simulink model "PID_2DOF"  (Simulink 7.0)
settings: Solver=ode3  StartTime=0.0  StopTime=10.0  RelTol=1e-3
undefined symbols (not defined in the file): Kd1, Kd2, Ki1, Ki2, Kp1, Kp2, L1, L2, M1, M2, theta1, theta2
settings Model: Creator=user  LastModifiedBy=user

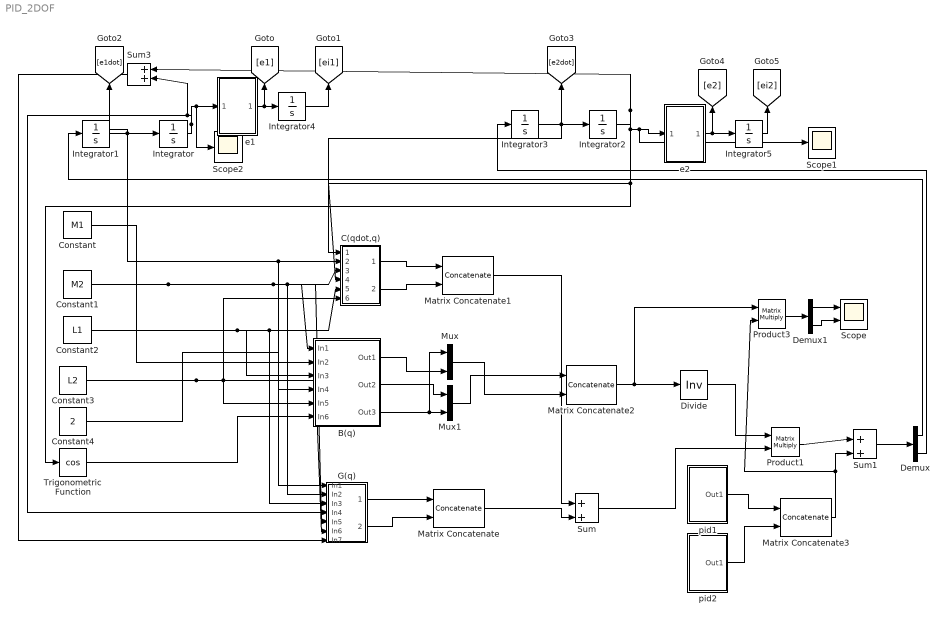
== system PID_2DOF ==
  B(q) : Subsystem
  C(qdot,q) : Subsystem
  Constant : Constant  Value=M1  OutDataType=sfix(16)  OutScaling=2^0
  Constant1 : Constant  Value=M2  OutDataType=sfix(16)  OutScaling=2^0
  Constant2 : Constant  Value=L1  OutDataType=sfix(16)  OutScaling=2^0
  Constant3 : Constant  Value=L2  OutDataType=sfix(16)  OutScaling=2^0
  Constant4 : Constant  Value=2  OutDataType=sfix(16)  OutScaling=2^0
  Demux : Demux  Outputs=2
  Demux1 : Demux  Outputs=2
  Divide : Product  Inputs=/  Multiplication=Matrix(*)  OutDataType=sfix(16)  OutScaling=2^-10
  G(q) : Subsystem
  Integrator{,1..5} (6 alike) : Integrator
  Matrix Concatenate : Concatenate  Mode=Vector  ConcatenateDimension=2
  Matrix Concatenate1 : Concatenate  Mode=Vector  ConcatenateDimension=2
  Matrix Concatenate2 : Concatenate  Mode=Multidimensional array  ConcatenateDimension=2
  Matrix Concatenate3 : Concatenate  Mode=Vector  ConcatenateDimension=2
  Mux : Mux  Inputs=2
  Mux1 : Mux  Inputs=2
  Product1 : Product  Multiplication=Matrix(*)  OutDataType=sfix(16)  OutScaling=2^0  RndMeth=Zero
  Product3 : Product  Multiplication=Matrix(*)  OutDataType=sfix(16)  OutScaling=2^0  RndMeth=Zero
  Scope : Scope  NumInputPorts=2
      settings: YMin=-5~-5  YMax=5~5
  Scope1 : Scope
  Scope2 : Scope
      settings: SaveName=ScopeData2
  Sum : Sum  Inputs=|++  OutDataType=sfix(16)  OutScaling=2^0
  Sum1 : Sum  Inputs=|++  OutDataType=sfix(16)  OutScaling=2^0
  Sum3 : Sum  Orientation=left  Inputs=|++  OutDataType=sfix(16)  OutScaling=2^0
  Trigonometric Function : Trigonometry  Operator=cos
  e1 : Subsystem
  e2 : Subsystem
  pid1 : Subsystem
  pid2 : Subsystem
  wires:
  Constant/1 -> B(q)/2(In2)
  Constant4/1 -> B(q)/4(In4)
  Constant1/1 -> B(q)/1(In1), C(qdot,q)/3(In3), G(q)/2(In2), G(q)/5(In5)
  Constant2/1 -> B(q)/3(In3), C(qdot,q)/5(In5), G(q)/3(In3)
  Constant3/1 -> B(q)/5(In5), C(qdot,q)/6(In6), G(q)/6(In6)
  Trigonometric Function/1 -> B(q)/6(In6)
  Integrator1/1 -> Integrator/1, C(qdot,q)/2(In2), G(q)/1(In1), [e1dot]
  Integrator3/1 -> Integrator2/1, C(qdot,q)/1(In1), [e2dot]
  Integrator2/1 -> Trigonometric Function/1, C(qdot,q)/4(In4), Sum3/1, e2/1(In1), Scope1/1
  Integrator/1 -> Sum3/2, G(q)/4(In4), e1/1(In1), Scope2/1
  Sum3/1 -> G(q)/7(In7)
  G(q)/1(Out1) -> Matrix Concatenate/1
  G(q)/2(Out2) -> Matrix Concatenate/2
  C(qdot,q)/1(Out1) -> Matrix Concatenate1/1
  C(qdot,q)/2(Out2) -> Matrix Concatenate1/2
  B(q)/1(Out1) -> Mux/2
  B(q)/3(Out3) -> Mux/1, Mux1/2
  B(q)/2(Out2) -> Mux1/1
  Mux1/1 -> Matrix Concatenate2/1
  Mux/1 -> Matrix Concatenate2/2
  Matrix Concatenate/1 -> Sum/2
  Matrix Concatenate1/1 -> Sum/1
  Matrix Concatenate2/1 -> Divide/1, Product3/1
  Divide/1 -> Product1/1
  Sum/1 -> Product1/2
  Product1/1 -> Sum1/1
  e1/1(Out1) -> Integrator4/1, [e1]
  e2/1(Out1) -> Integrator5/1, [e2]
  Integrator4/1 -> [ei1]
  Integrator5/1 -> [ei2]
  pid1/1(Out1) -> Matrix Concatenate3/1
  pid2/1(Out1) -> Matrix Concatenate3/2
  Matrix Concatenate3/1 -> Sum1/2, Product3/2
  Sum1/1 -> Demux/1
  Demux/1 -> Integrator1/1
  Demux/2 -> Integrator3/1
  Product3/1 -> Demux1/1
  Demux1/1 -> Scope/1
  Demux1/2 -> Scope/2

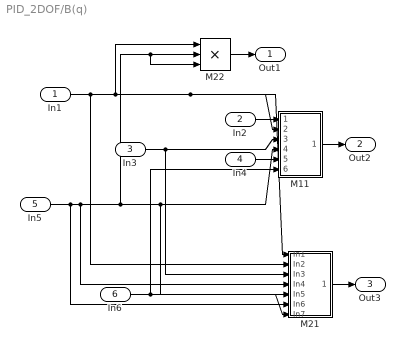
== system PID_2DOF/B(q) ==
  In1 : Inport
  In2 : Inport  Port=2
  In3 : Inport  Port=3
  In4 : Inport  Port=4
  In5 : Inport  Port=5
  In6 : Inport  Port=6
  M11 : Subsystem
  M21 : Subsystem
  M22 : Product  Inputs=3  OutDataType=sfix(16)  OutScaling=2^0  RndMeth=Zero
  Out1 : Outport
  Out2 : Outport  Port=2
  Out3 : Outport  Port=3
  wires:
  In6/1 -> M21/7(In7), M11/6(In6)
  In1/1 -> M22/1, M21/1(In1), M11/2(In2), M21/2(In2)
  In3/1 -> M21/3(In3), M11/3(In3)
  In5/1 -> M21/6(In6), M22/3, M22/2, M21/5(In5), M11/4(In4), M21/4(In4)
  M22/1 -> Out1/1
  In2/1 -> M11/1(In1)
  M11/1(Out1) -> Out2/1
  In4/1 -> M11/5(In5)
  M21/1(Out1) -> Out3/1

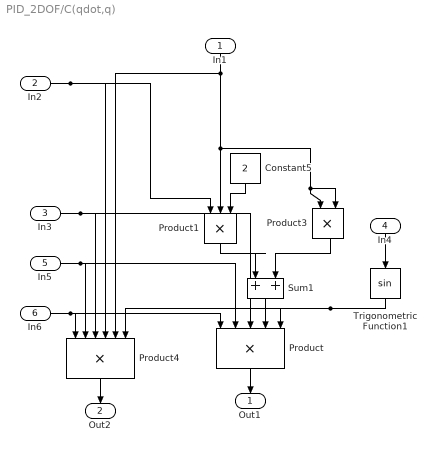
== system PID_2DOF/C(qdot,q) ==
  In1 : Inport  Orientation=down
  In2 : Inport  Port=2
  In3 : Inport  Port=3
  In4 : Inport  Orientation=down  Port=4
  In5 : Inport  Port=5
  In6 : Inport  Port=6
  Constant5 : Constant  Orientation=down  Value=2  OutDataType=sfix(16)  OutScaling=2^0
  Product : Product  Orientation=down  Inputs=5  OutDataType=sfix(16)  OutScaling=2^0  RndMeth=Zero
  Product1 : Product  Orientation=down  Inputs=3  OutDataType=sfix(16)  OutScaling=2^0  RndMeth=Zero
  Product3 : Product  Orientation=down  OutDataType=sfix(16)  OutScaling=2^0  RndMeth=Zero
  Product4 : Product  Orientation=down  Inputs=6  OutDataType=sfix(16)  OutScaling=2^0  RndMeth=Zero
  Sum1 : Sum  Orientation=down  Inputs=|++  OutDataType=sfix(16)  OutScaling=2^0
  Trigonometric Function1 : Trigonometry  Orientation=down
  Out1 : Outport  Orientation=down
  Out2 : Outport  Orientation=down  Port=2
  wires:
  Constant5/1 -> Product1/3
  Product3/1 -> Sum1/2
  Product1/1 -> Sum1/1
  Sum1/1 -> Product/4
  Trigonometric Function1/1 -> Product/5, Product4/6
  In1/1 -> Product1/2, Product3/1, Product3/2, Product4/5
  In2/1 -> Product1/1, Product4/4
  In3/1 -> Product/3, Product4/3
  In4/1 -> Trigonometric Function1/1
  In5/1 -> Product/2, Product4/2
  In6/1 -> Product/1, Product4/1
  Product/1 -> Out1/1
  Product4/1 -> Out2/1

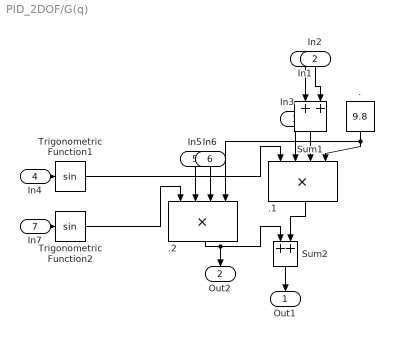
== system PID_2DOF/G(q) ==
  In1 : Inport  Orientation=down
  In2 : Inport  Orientation=down  Port=2
  In3 : Inport  Orientation=down  Port=3
  In4 : Inport  Port=4
  In5 : Inport  Orientation=down  Port=5
  In6 : Inport  Orientation=down  Port=6
  In7 : Inport  Port=7
  . : Constant  Orientation=down  Value=9.8  OutDataType=sfix(16)  OutScaling=2^0
  .1 : Product  Orientation=down  Inputs=4  OutDataType=sfix(16)  OutScaling=2^0  RndMeth=Zero
  .2 : Product  Orientation=down  Inputs=4  OutDataType=sfix(16)  OutScaling=2^0  RndMeth=Zero
  Sum1 : Sum  Orientation=down  Inputs=|++  OutDataType=sfix(16)  OutScaling=2^0
  Sum2 : Sum  Orientation=down  Inputs=|++  OutDataType=sfix(16)  OutScaling=2^0
  Trigonometric Function1 : Trigonometry
  Trigonometric Function2 : Trigonometry
  Out1 : Outport  Orientation=down
  Out2 : Outport  Orientation=down  Port=2
  wires:
  ./1 -> .1/4, .2/4
  Sum1/1 -> .1/3
  Trigonometric Function1/1 -> .1/1
  Trigonometric Function2/1 -> .2/1
  .2/1 -> Sum2/1, Out2/1
  .1/1 -> Sum2/2
  In1/1 -> Sum1/1
  In2/1 -> Sum1/2
  In3/1 -> .1/2
  In4/1 -> Trigonometric Function1/1
  In5/1 -> .2/2
  In6/1 -> .2/3
  In7/1 -> Trigonometric Function2/1
  Sum2/1 -> Out1/1

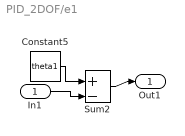
== system PID_2DOF/e1 ==
  In1 : Inport
  Constant5 : Constant  Value=theta1  OutDataType=sfix(16)  OutScaling=2^0
  Sum2 : Sum  Inputs=|+-  OutDataType=sfix(16)  OutScaling=2^0
  Out1 : Outport
  wires:
  Constant5/1 -> Sum2/1
  In1/1 -> Sum2/2
  Sum2/1 -> Out1/1

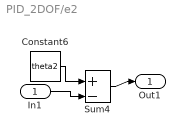
== system PID_2DOF/e2 ==
  In1 : Inport
  Constant6 : Constant  Value=theta2  OutDataType=sfix(16)  OutScaling=2^0
  Sum4 : Sum  Inputs=|+-  OutDataType=sfix(16)  OutScaling=2^0
  Out1 : Outport
  wires:
  Constant6/1 -> Sum4/1
  In1/1 -> Sum4/2
  Sum4/1 -> Out1/1

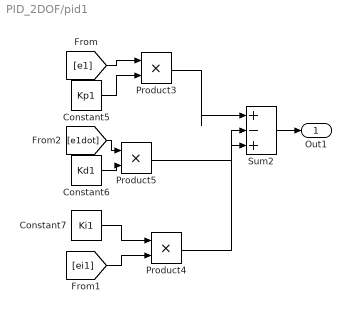
== system PID_2DOF/pid1 ==
  Constant5 : Constant  Value=Kp1  OutDataType=sfix(16)  OutScaling=2^0
  Constant6 : Constant  Value=Kd1  OutDataType=sfix(16)  OutScaling=2^0
  Constant7 : Constant  Value=Ki1  OutDataType=sfix(16)  OutScaling=2^0
  Product3 : Product  OutDataType=sfix(16)  OutScaling=2^0  RndMeth=Zero
  Product4 : Product  OutDataType=sfix(16)  OutScaling=2^0  RndMeth=Zero
  Product5 : Product  OutDataType=sfix(16)  OutScaling=2^0  RndMeth=Zero
  Sum2 : Sum  Inputs=|+-+  OutDataType=sfix(16)  OutScaling=2^0
  Out1 : Outport
  wires:
  [e1] -> Product3/1
  Constant5/1 -> Product3/2
  Constant7/1 -> Product4/1
  [ei1] -> Product4/2
  [e1dot] -> Product5/1
  Constant6/1 -> Product5/2
  Product3/1 -> Sum2/1
  Product5/1 -> Sum2/2
  Product4/1 -> Sum2/3
  Sum2/1 -> Out1/1

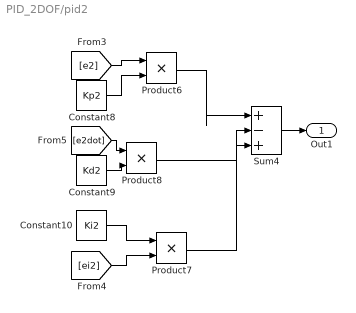
== system PID_2DOF/pid2 ==
  Constant10 : Constant  Value=Ki2  OutDataType=sfix(16)  OutScaling=2^0
  Constant8 : Constant  Value=Kp2  OutDataType=sfix(16)  OutScaling=2^0
  Constant9 : Constant  Value=Kd2  OutDataType=sfix(16)  OutScaling=2^0
  Product6 : Product  OutDataType=sfix(16)  OutScaling=2^0  RndMeth=Zero
  Product7 : Product  OutDataType=sfix(16)  OutScaling=2^0  RndMeth=Zero
  Product8 : Product  OutDataType=sfix(16)  OutScaling=2^0  RndMeth=Zero
  Sum4 : Sum  Inputs=|+-+  OutDataType=sfix(16)  OutScaling=2^0
  Out1 : Outport
  wires:
  Product6/1 -> Sum4/1
  Product8/1 -> Sum4/2
  Product7/1 -> Sum4/3
  Constant9/1 -> Product8/2
  [e2dot] -> Product8/1
  [ei2] -> Product7/2
  Constant10/1 -> Product7/1
  Constant8/1 -> Product6/2
  [e2] -> Product6/1
  Sum4/1 -> Out1/1

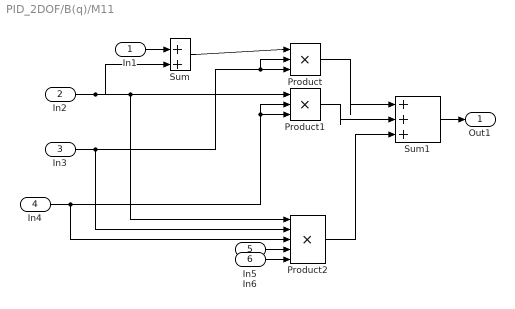
== system PID_2DOF/B(q)/M11 ==
  In1 : Inport
  In2 : Inport  Port=2
  In3 : Inport  Port=3
  In4 : Inport  Port=4
  In5 : Inport  Port=5
  In6 : Inport  Port=6
  Product : Product  Inputs=3  OutDataType=sfix(16)  OutScaling=2^0  RndMeth=Zero
  Product1 : Product  Inputs=3  OutDataType=sfix(16)  OutScaling=2^0  RndMeth=Zero
  Product2 : Product  Inputs=5  OutDataType=sfix(16)  OutScaling=2^0  RndMeth=Zero
  Sum : Sum  Inputs=|++  OutDataType=sfix(16)  OutScaling=2^0
  Sum1 : Sum  Inputs=|+++  OutDataType=sfix(16)  OutScaling=2^0
  Out1 : Outport
  wires:
  In2/1 -> Product2/1, Product1/1, Sum/2
  Sum/1 -> Product/1
  In3/1 -> Product2/2, Product/2, Product/3
  In4/1 -> Product2/3, Product1/3, Product1/2
  Product/1 -> Sum1/1
  Product1/1 -> Sum1/2
  Product2/1 -> Sum1/3
  In1/1 -> Sum/1
  Sum1/1 -> Out1/1
  In5/1 -> Product2/4
  In6/1 -> Product2/5

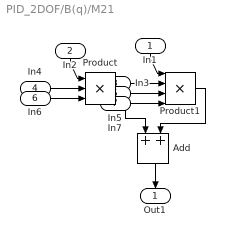
== system PID_2DOF/B(q)/M21 ==
  In1 : Inport  Orientation=down
  In2 : Inport  Orientation=down  Port=2
  In3 : Inport  Port=3
  In4 : Inport  Port=4
  In5 : Inport  Port=5
  In6 : Inport  Port=6
  In7 : Inport  Port=7
  Add : Sum  Orientation=down  OutDataType=sfix(16)  OutScaling=2^-10
  Product : Product  Inputs=3  OutDataType=sfix(16)  OutScaling=2^0  RndMeth=Zero
  Product1 : Product  Inputs=4  OutDataType=sfix(16)  OutScaling=2^0  RndMeth=Zero
  Out1 : Outport  Orientation=down
  wires:
  Product/1 -> Add/1
  Product1/1 -> Add/2
  In1/1 -> Product1/1
  In2/1 -> Product/1
  In3/1 -> Product1/2
  In4/1 -> Product/2
  In5/1 -> Product1/3
  In6/1 -> Product/3
  In7/1 -> Product1/4
  Add/1 -> Out1/1
